simulink model "JointSpaceInverseDynamic"  (R2020b)
settings: Solver=VariableStepAuto  StartTime=0.0  StopTime=5  RelTol=1e-3
values from neighbouring files (symbols this model uses):
  KD = diag([ 40  40  40])    [parameters.m]
  KP = diag([500 500 500])    [parameters.m]
libraries: vrlib x1
settings Model: Creator=Edoardo  LastModifiedBy=Edoardo

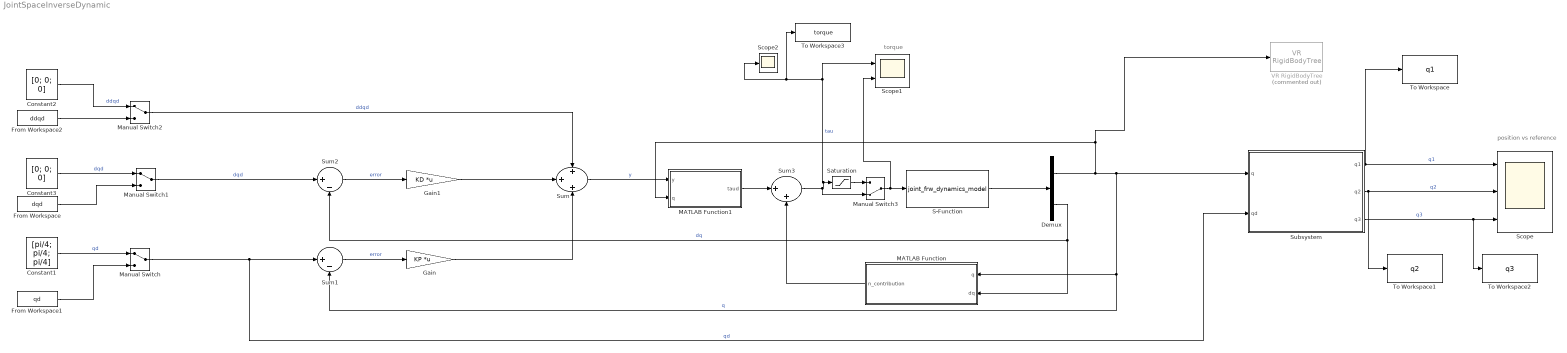
== system JointSpaceInverseDynamic ==
  note: torque
  note: position vs reference
  Constant1 : Constant  Value=[pi/4; pi/4; pi/4]  VectorParams1D=off
  Constant2 : Constant  Value=[0; 0; 0]  VectorParams1D=off
  Constant3 : Constant  Value=[0; 0; 0]  VectorParams1D=off
  Demux : Demux  Outputs=2
  From Workspace : FromWorkspace  VariableName=dqd
  From Workspace1 : FromWorkspace  VariableName=qd
  From Workspace2 : FromWorkspace  VariableName=ddqd
  Gain : Gain  Gain=KP  Multiplication=Matrix(K*u) (u vector)
  Gain1 : Gain  Gain=KD  Multiplication=Matrix(K*u) (u vector)
  MATLAB Function : MATLAB Function  TreatAsAtomicUnit=on
  MATLAB Function1 : MATLAB Function  TreatAsAtomicUnit=on
  Manual Switch : ManualSwitch
  Manual Switch1 : ManualSwitch
  Manual Switch2 : ManualSwitch
  Manual Switch3 : ManualSwitch  CurrentSetting=0
  S-Function : S-Function  FunctionName=joint_frw_dynamics_model  Parameters=myRobot  SFunctionDeploymentMode=off  EnableBusSupport=off
  Saturation : Saturate
  Scope : Scope  NumInputPorts=3
  Scope1 : Scope  NumInputPorts=2
  Scope2 : Scope
  Subsystem : Subsystem
  Sum : Sum  Inputs=+++
  Sum1 : Sum  Inputs=|+-
  Sum2 : Sum  Inputs=|+-
  Sum3 : Sum  Inputs=|++
  To Workspace : ToWorkspace  VariableName=q1  SaveFormat=Timeseries  SampleTime=-1
  To Workspace1 : ToWorkspace  VariableName=q2  SaveFormat=Timeseries  SampleTime=-1
  To Workspace2 : ToWorkspace  VariableName=q3  SaveFormat=Timeseries  SampleTime=-1
  To Workspace3 : ToWorkspace  VariableName=torque  SaveFormat=Timeseries  SampleTime=-1
  VR RigidBodyTree : vrlib/VR RigidBodyTree  Commented=on  RBT=robot  useRBT=on  Ts=-1  ForceViewerOpen=on
      settings: SourceProductBaseCode=SL
  wires:
  Gain1/1 -> Sum/2
  Gain/1 -> Sum/3
  Sum2/1 -> Gain1/1  "error"
  Sum1/1 -> Gain/1  "error"
  S-Function/1 -> Demux/1
  Sum3/1 -> Manual Switch3/2, Scope1/1, To Workspace3/1, Scope2/1, Saturation/1  "tau"
  MATLAB Function/1(n_contribution) -> Sum3/2
  MATLAB Function1/1(taud) -> Sum3/1
  Sum/1 -> MATLAB Function1/1(y)  "y"
  Manual Switch2/1 -> Sum/1  "ddqd"
  Demux/2 -> MATLAB Function/2(dq), Sum2/2  "dq"
  Manual Switch1/1 -> Sum2/1  "dqd"
  Manual Switch/1 -> Subsystem/2(qd), Sum1/1  "qd"
  Constant1/1 -> Manual Switch/1  "qd"
  Constant3/1 -> Manual Switch1/1  "dqd"
  Constant2/1 -> Manual Switch2/1  "ddqd"
  From Workspace2/1 -> Manual Switch2/2
  From Workspace/1 -> Manual Switch1/2
  From Workspace1/1 -> Manual Switch/2
  Demux/1 -> VR RigidBodyTree/1, MATLAB Function1/2(q), Subsystem/1(q), MATLAB Function/1(q), Sum1/2  "q"
  Manual Switch3/1 -> Scope1/2, S-Function/1
  Saturation/1 -> Manual Switch3/1
  Subsystem/2(q2) -> Scope/2, To Workspace1/1  "q2"
  Subsystem/1(q1) -> To Workspace/1, Scope/1  "q1"
  Subsystem/3(q3) -> Scope/3, To Workspace2/1  "q3"

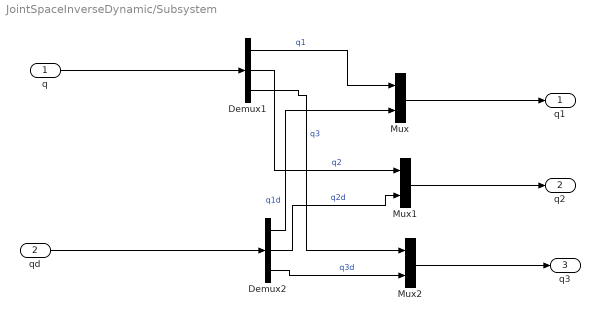
== system JointSpaceInverseDynamic/Subsystem ==
  q : Inport
  qd : Inport  Port=2
  Demux1 : Demux  Outputs=3
  Demux2 : Demux  Outputs=3
  Mux : Mux  Inputs=2
  Mux1 : Mux  Inputs=2
  Mux2 : Mux  Inputs=2
  q1 : Outport
  q2 : Outport  Port=2
  q3 : Outport  Port=3
  wires:
  Demux2/2 -> Mux1/2  "q2d"
  Mux2/1 -> q3/1
  Mux1/1 -> q2/1
  Demux2/1 -> Mux/2  "q1d"
  Demux1/2 -> Mux1/1  "q2"
  Demux1/1 -> Mux/1  "q1"
  Demux1/3 -> Mux2/1  "q3"
  Demux2/3 -> Mux2/2  "q3d"
  Mux/1 -> q1/1
  q/1 -> Demux1/1
  qd/1 -> Demux2/1

== matlab function JointSpaceInverseDynamic/MATLAB Function ==
  data: q input size=3; n_contribution output; dq input size=3
function n_contribution = n(q,dq)
    n_contribution = getCHatLagrangian(q,dq)*dq + getGHatLagrangian(q);

== matlab function JointSpaceInverseDynamic/MATLAB Function1 ==
  data: y input; taud output; q input size=3
function taud = B(y, q)

    
 taud = getBHatLagrangian(q)*y;
%taud = y;
